simulink model "my_system"  (R2020a)
settings: Solver=VariableStepAuto  StartTime=0.0  StopTime=10.0  RelTol=1e-3
settings Model: Creator=User  LastModifiedBy=User

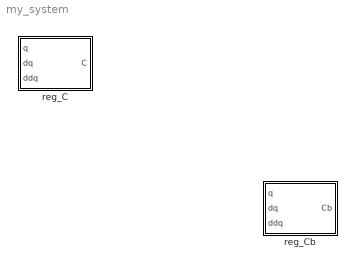
== system my_system ==
  reg_C : MATLAB Function  TreatAsAtomicUnit=on
  reg_Cb : MATLAB Function  TreatAsAtomicUnit=on

== matlab function my_system/reg_Cb ==
  data: q input; Cb output; dq input; ddq input
function Cb = reg_Cb(q,dq,ddq)
%#codegen

%    This function was generated by the Symbolic Math Toolbox version 8.5.
%    15-Nov-2022 11:13:43
ddq1 = ddq(1);
ddq2 = ddq(2);
dq1  = dq(1);
dq2  = dq(2);
q1   = q(1);
q2   = q(2);

t2 = cos(q2);
t3 = sin(q2);
t4 = ddq1+ddq2;
t5 = dq1+dq2;
t6 = q1+q2;
t7 = ddq1.*t2;
t8 = cos(t6);
t9 = ddq1.*t3;
t10 = sin(t6);
t11 = dq1.*dq2.*t3;
t12 = dq1.*dq2.*t2;
t13 = -t9;
t14 = -t11;
t15 = -t12;
t16 = t8.*(9.81e+2./1.0e+2);
t17 = t10.*(9.81e+2./1.0e+2);
t18 = -t17;
Cb = reshape([ddq1,0.0,cos(q1).*(9.81e+2./1.0e+2),0.0,sin(q1).*(-9.81e+2./1.0e+2),0.0,t4,t4,t7+t14+t16+t2.*t4-dq2.*t3.*t5,t7+t14+t16+dq1.*t3.*t5,t13+t15+t18-t3.*t4-dq2.*t2.*t5,t13+t15+t18+dq1.*t2.*t5],[2,6]);

== matlab function my_system/reg_C ==
  data: q input; C output; dq input; ddq input
function C = reg_C(q,dq,ddq)
%#codegen

%    This function was generated by the Symbolic Math Toolbox version 8.5.
%    15-Nov-2022 11:13:43
ddq1 = ddq(1);
ddq2 = ddq(2);
dq1  = dq(1);
dq2  = dq(2);
q1   = q(1);
q2   = q(2);

t2 = cos(q1);
t3 = cos(q2);
t4 = sin(q2);
t5 = ddq1+ddq2;
t6 = dq1+dq2;
t7 = q1+q2;
t8 = ddq1.*t3;
t9 = cos(t7);
t10 = ddq1.*t4;
t11 = sin(t7);
t12 = dq1.*dq2.*t4;
t13 = dq1.*dq2.*t3;
t17 = t2.*(9.81e+2./1.0e+2);
t14 = -t10;
t15 = -t12;
t16 = -t13;
t18 = t9.*(9.81e+2./1.0e+2);
t19 = t11.*(9.81e+2./1.0e+2);
t20 = -t19;
C = reshape([0.0,0.0,0.0,0.0,0.0,0.0,0.0,0.0,0.0,0.0,ddq1,0.0,t17,0.0,sin(q1).*(-9.81e+2./1.0e+2),0.0,0.0,0.0,0.0,0.0,0.0,0.0,0.0,0.0,0.0,0.0,0.0,0.0,0.0,0.0,t5,t5,t8+t15+t18+t3.*t5-dq2.*t4.*t6,t8+t15+t18+dq1.*t4.*t6,t14+t16+t20-t4.*t5-dq2.*t3.*t6,t14+t16+t20+dq1.*t3.*t6,0.0,0.0,ddq1+t17,0.0],[2,20]);
